simulink model "ex2"  (R2021b)
settings: Solver=VariableStepAuto  StartTime=0.0  StopTime=40.0  RelTol=1e-3
settings SolverCC: AlgebraicLoopSolver=TrustRegion
settings DebuggingCC: SFMachineParentedDataDiag=warning

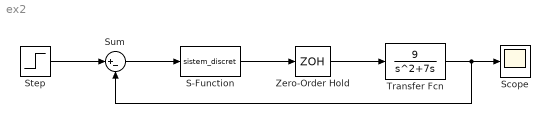
== system ex2 ==
  S-Function : S-Function  FunctionName=sistem_discret  Parameters=fi,gama,C_1, D_1  SFunctionDeploymentMode=off  EnableBusSupport=off
  Scope : Scope
  Step : Step  SampleTime=0.1
  Sum : Sum  Inputs=|+-  SampleTime=0.1
  Transfer Fcn : TransferFcn  Numerator=[9]  Denominator=[1 7 0]
  Zero-Order Hold : ZeroOrderHold  SampleTime=-1
  wires:
  Step/1 -> Sum/1
  Sum/1 -> S-Function/1
  S-Function/1 -> Zero-Order Hold/1
  Zero-Order Hold/1 -> Transfer Fcn/1
  Transfer Fcn/1 -> Sum/2, Scope/1
